simulink model "TesteEloGhendy"  (R2021b)
settings: Solver=FixedStepAuto  StartTime=0.0  StopTime=TempoSimulacao  RelTol=1e-3
values from neighbouring files (symbols this model uses):
  FatorSimulacao = 1e-3    (= 0.001)    [TesteRealCurtoFuses.m]    (also in TesteRealCurto_SemFuse.m)
  le = 1e-10    [TesteRealCurto.m]    (also in TesteRealCurtoFuses.m; TesteRealCurto_SemFuse.m)
  lm = (imag(Zm)/(2*pi*f))*d    [TesteRealCurto.m]    (also in TesteRealCurtoFuses.m; TesteRealCurto_SemFuse.m)
  lp = (imag(Zp)/(2*pi*f))*d    [TesteRealCurto.m]    (also in TesteRealCurtoFuses.m; TesteRealCurto_SemFuse.m)
  NRE = 1e-12    [TesteRealCurto.m]    (also in TesteRealCurtoFuses.m; TesteRealCurto_SemFuse.m)
  rm = real(Zm)*d    [TesteRealCurto.m]    (also in TesteRealCurtoFuses.m; TesteRealCurto_SemFuse.m)
  rp = real(Zp)*d    [TesteRealCurto.m]    (also in TesteRealCurtoFuses.m; TesteRealCurto_SemFuse.m)
  rtc = 10    [TesteRealCurto.m]    (also in TesteRealCurtoFuses.m; TesteRealCurto_SemFuse.m)
  rti = 10    [TesteRealCurto.m]    (also in TesteRealCurtoFuses.m; TesteRealCurto_SemFuse.m)
undefined symbols (not defined in the file or in its folder): D11, Delta, POT, PotConsumidor, Ra_Curto, Rb_Curto, Rc_Curto
libraries: spsRMSLib x15, spsBreakerLib x7, spsCurrentMeasurementLib x7, spsSeriesRLCBranchLib x6, spsThreePhaseVIMeasurementLib x4, spsThreePhaseTransformerTwoWindingsLib x2, spsThreePhaseSeriesRLCLoadLib x1, spsThreePhaseBreakerLib x1, spsThreePhaseSourceLib x1, spsMutualInductanceLib x1, spspowerguiLib x1
(part 1 of 2)
settings Model: Creator=USER  LastModifiedBy=Leonardo-Felipe
settings SolverCC: ZeroCrossAlgorithm=Adaptive
settings DebuggingCC: MaskedZcDiagnostic=none  IgnoredZcDiagnostic=none

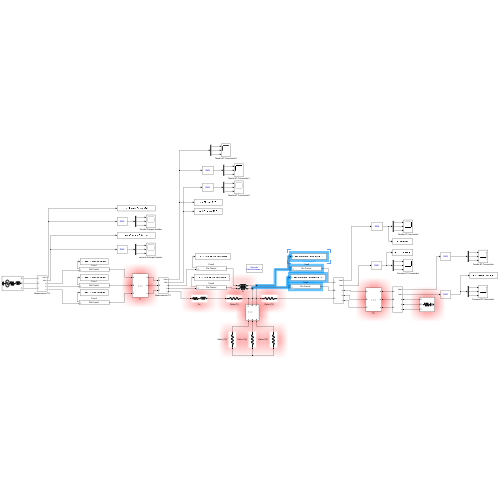
[thumbnail: Simulink's stored preview of the top-level diagram]
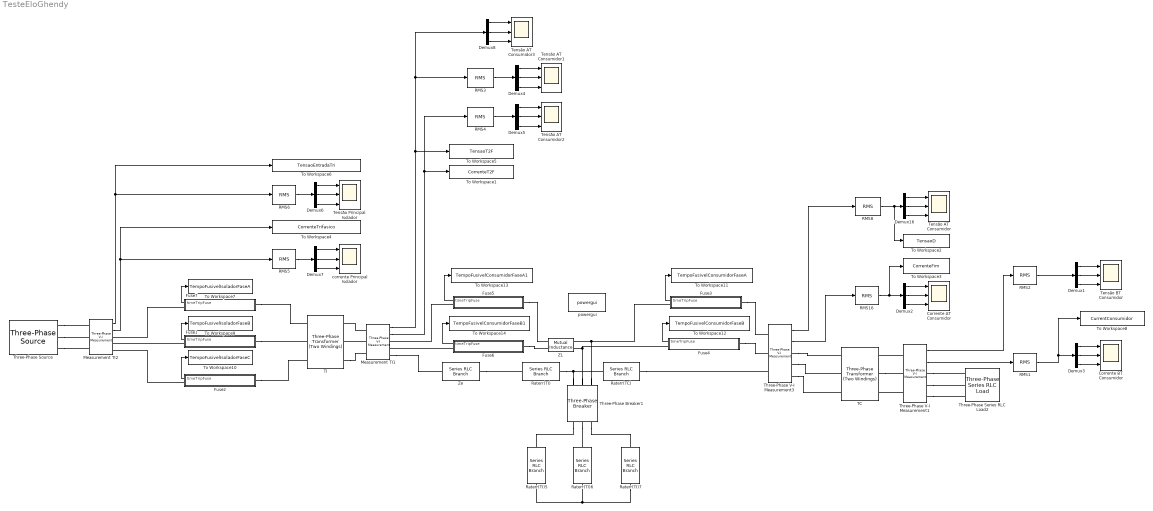
== system TesteEloGhendy ==
  Corrente AT Consumidor : Scope  NumInputPorts=3
  Corrente BT Consumidor : Scope  NumInputPorts=3
  Demux{1..8,16} (9 alike) : Demux  Outputs=3
  Fuse1 : Subsystem  mask{tipofuse=15K, a=346.4070, b=-257.6697, c=71.6644, d=-8.8225, e=0.4027, IoTot=15}
      mask prompts: tipofuse "Tipo de Fusivel"
      mask TypeOptions tipofuse: 15K
      mask Callback tipofuse:
      | switch(get_param(gcb,'tipofuse'))
      |     case '1H'
      |         set_param(gcb,'a','11.5834');
      |         set_param(gcb,'b','-7.7159');
      |         set_param(gcb,'c','2.2435');
      |         set_param(gcb,'d','-0.4141');
      |         set_param(gcb,'e','0.0293');
      |         set_param(gcb,'IoTot','1');
      |     case '2H'
      |         set_param(gcb,'a','15.3612');
      |         set_param(gcb,'b','-11.3048');
      |         set_param(gcb,'c','3.7855');
      |         set_param(gcb,'d','-0.6767');
      |         set_param(gcb,'e','0.0442');
      |         set_param(gcb,'IoTot','2');
      |     case '3H'
      |         set_param(gcb,'a','16.6469');
      |         set_param(gcb,'b','-10.3608');
      |         set_param(gcb,'c','2.8987');
      |         set_param(gcb,'d','-0.4844');
      |         set_param(gcb,'e','0.0315');
      |         set_param(gcb,'IoTot','3');
      |     case '5H'
      |         set_param(gcb,'a','33.5364');
      |         set_param(gcb,'b','-24.1389');
      |         set_param(gcb,'c','7.0071');
      |         set_param(gcb,'d','-1.0167');
      |         set_param(gcb,'e','0.0569');
      |         set_param(gcb,'IoTot','5');
      |     case '8H'
      |         set_param(gcb,'a','137.5572');
      |         set_param(gcb,'b','-119.0117');
      |         set_param(gcb,'c','38.2794');
      |         set_param(gcb,'d','-5.4440');
      |         set_param(gcb,'e','0.2846');
      |         set_param(gcb,'IoTot','8');
      |     case '6K'
      |         set_param(gcb,'a','181.2568');
      |         set_param(gcb,'b','-167.5711');
      |         set_param(gcb,'c','57.6673');
      |         set_param(gcb,'d','-8.7672');
      |         set_param(gcb,'e','0.4916');
      |         set_param(gcb,'IoTot','6');
      |     case '8K'
      |         set_param(gcb,'a','201.6778');
      |         set_param(gcb,'b','-175.2376');
      |         set_param(gcb,'c','56.8760');
      |         set_param(gcb,'d','-8.1725');
      |         set_param(gcb,'e','0.4340');
      |         set_param(gcb,'IoTot','8');
      |     case '10K'
      |         set_param(gcb,'a','251.8801');
      |         set_param(gcb,'b','-206.6378');
      |         set_param(gcb,'c','63.3069');
      |         set_param(gcb,'d','-8.5810');
      |         set_param(gcb,'e','0.4304');
      |         set_param(gcb,'IoTot','10');
      |     case '12K'
      |         set_param(gcb,'a','294.2461');
      |         set_param(gcb,'b','-229.0340');
      |         set_param(gcb,'c','66.6693');
      |         set_param(gcb,'d','-8.5945');
      |         set_param(gcb,'e','0.4107');
      |         set_param(gcb,'IoTot','12');
      |     case '15K'
      |         set_param(gcb,'a','346.4070');
      |         set_param(gcb,'b','-257.6697');
      |         set_param(gcb,'c','71.6644');
      |         set_param(gcb,'d','-8.8225');
      |         set_param(gcb,'e','0.4027');
      |         set_param(gcb,'IoTot','15');
      |     case '20K'
      |         set_param(gcb,'a','382.4620');
      |         set_param(gcb,'b','-271.3985');
      |         set_param(gcb,'c','72.1161');
      |         set_param(gcb,'d','-8.4924');
      |         set_param(gcb,'e','0.3714');
      |         set_param(gcb,'IoTot','20');
      |     case '25K'
      |         set_param(gcb,'a','469.9755');
      |         set_param(gcb,'b','-321.2512');
      |         set_param(gcb,'c','82.1749');
      |         set_param(gcb,'d','-9.3092');
      |         set_param(gcb,'e','0.3918');
      |         set_param(gcb,'IoTot','25');
      |     case '30K'
      |         set_param(gcb,'a','516.7220');
      |         set_param(gcb,'b','-337.6034');
      |         set_param(gcb,'c','82.5876');
      |         set_param(gcb,'d','-8.9522');
      |         set_param(gcb,'e','0.3608');
      |         set_param(gcb,'IoTot','30');
      |     case '40K'
      |         set_param(gcb,'a','672.1360');
      |         set_param(gcb,'b','-424.7867');
      |         set_param(gcb,'c','100.3706');
      |         set_param(gcb,'d','-10.4950');
      |         set_param(gcb,'e','0.4080');
      |         set_param(gcb,'IoTot','40');
      |     case '50K'
      |         set_param(gcb,'a','691.3953');
      |         set_param(gcb,'b','-419.2300');
      |         set_param(gcb,'c','95.1730');
      |         set_param(gcb,'d','-9.5735');
      |         set_param(gcb,'e','0.3584');
      |         set_param(gcb,'IoTot','50');
      |     case '65K'
      |         set_param(gcb,'a','841.8993');
      |         set_param(gcb,'b','-492.8148');
      |         set_param(gcb,'c','107.9499');
      |         set_param(gcb,'d','-10.4731');
      |         set_param(gcb,'e','0.3783');
      |         set_param(gcb,'IoTot','65');
      |     case '80K'
      |         set_param(gcb,'a','881.1649');
      |         set_param(gcb,'b','-499.4578');
      |         set_param(gcb,'c','106.0005');
      |         set_param(gcb,'d','-9.9685');
      |         set_param(gcb,'e','0.3492');
      |         set_param(gcb,'IoTot','80');
      |     case '100K'
      |         set_param(gcb,'a','1020.0325');
      |         set_param(gcb,'b','-554.4466');
      |         set_param(gcb,'c','112.8674');
      |         set_param(gcb,'d','-10.1845');
      |         set_param(gcb,'e','0.3425');
      |         set_param(gcb,'IoTot','100');
      | end
      mask Display: disp('Elo Fusivel');
  Fuse2 : Subsystem  mask{tipofuse=15K, a=346.4070, b=-257.6697, c=71.6644, d=-8.8225, e=0.4027, IoTot=15}
      mask prompts: tipofuse "Tipo de Fusivel"
      mask TypeOptions tipofuse: 15K
      mask Callback tipofuse:
      | switch(get_param(gcb,'tipofuse'))
      |     case '1H'
      |         set_param(gcb,'a','11.5834');
      |         set_param(gcb,'b','-7.7159');
      |         set_param(gcb,'c','2.2435');
      |         set_param(gcb,'d','-0.4141');
      |         set_param(gcb,'e','0.0293');
      |         set_param(gcb,'IoTot','1');
      |     case '2H'
      |         set_param(gcb,'a','15.3612');
      |         set_param(gcb,'b','-11.3048');
      |         set_param(gcb,'c','3.7855');
      |         set_param(gcb,'d','-0.6767');
      |         set_param(gcb,'e','0.0442');
      |         set_param(gcb,'IoTot','2');
      |     case '3H'
      |         set_param(gcb,'a','16.6469');
      |         set_param(gcb,'b','-10.3608');
      |         set_param(gcb,'c','2.8987');
      |         set_param(gcb,'d','-0.4844');
      |         set_param(gcb,'e','0.0315');
      |         set_param(gcb,'IoTot','3');
      |     case '5H'
      |         set_param(gcb,'a','33.5364');
      |         set_param(gcb,'b','-24.1389');
      |         set_param(gcb,'c','7.0071');
      |         set_param(gcb,'d','-1.0167');
      |         set_param(gcb,'e','0.0569');
      |         set_param(gcb,'IoTot','5');
      |     case '8H'
      |         set_param(gcb,'a','137.5572');
      |         set_param(gcb,'b','-119.0117');
      |         set_param(gcb,'c','38.2794');
      |         set_param(gcb,'d','-5.4440');
      |         set_param(gcb,'e','0.2846');
      |         set_param(gcb,'IoTot','8');
      |     case '6K'
      |         set_param(gcb,'a','181.2568');
      |         set_param(gcb,'b','-167.5711');
      |         set_param(gcb,'c','57.6673');
      |         set_param(gcb,'d','-8.7672');
      |         set_param(gcb,'e','0.4916');
      |         set_param(gcb,'IoTot','6');
      |     case '8K'
      |         set_param(gcb,'a','201.6778');
      |         set_param(gcb,'b','-175.2376');
      |         set_param(gcb,'c','56.8760');
      |         set_param(gcb,'d','-8.1725');
      |         set_param(gcb,'e','0.4340');
      |         set_param(gcb,'IoTot','8');
      |     case '10K'
      |         set_param(gcb,'a','251.8801');
      |         set_param(gcb,'b','-206.6378');
      |         set_param(gcb,'c','63.3069');
      |         set_param(gcb,'d','-8.5810');
      |         set_param(gcb,'e','0.4304');
      |         set_param(gcb,'IoTot','10');
      |     case '12K'
      |         set_param(gcb,'a','294.2461');
      |         set_param(gcb,'b','-229.0340');
      |         set_param(gcb,'c','66.6693');
      |         set_param(gcb,'d','-8.5945');
      |         set_param(gcb,'e','0.4107');
      |         set_param(gcb,'IoTot','12');
      |     case '15K'
      |         set_param(gcb,'a','346.4070');
      |         set_param(gcb,'b','-257.6697');
      |         set_param(gcb,'c','71.6644');
      |         set_param(gcb,'d','-8.8225');
      |         set_param(gcb,'e','0.4027');
      |         set_param(gcb,'IoTot','15');
      |     case '20K'
      |         set_param(gcb,'a','382.4620');
      |         set_param(gcb,'b','-271.3985');
      |         set_param(gcb,'c','72.1161');
      |         set_param(gcb,'d','-8.4924');
      |         set_param(gcb,'e','0.3714');
      |         set_param(gcb,'IoTot','20');
      |     case '25K'
      |         set_param(gcb,'a','469.9755');
      |         set_param(gcb,'b','-321.2512');
      |         set_param(gcb,'c','82.1749');
      |         set_param(gcb,'d','-9.3092');
      |         set_param(gcb,'e','0.3918');
      |         set_param(gcb,'IoTot','25');
      |     case '30K'
      |         set_param(gcb,'a','516.7220');
      |         set_param(gcb,'b','-337.6034');
      |         set_param(gcb,'c','82.5876');
      |         set_param(gcb,'d','-8.9522');
      |         set_param(gcb,'e','0.3608');
      |         set_param(gcb,'IoTot','30');
      |     case '40K'
      |         set_param(gcb,'a','672.1360');
      |         set_param(gcb,'b','-424.7867');
      |         set_param(gcb,'c','100.3706');
      |         set_param(gcb,'d','-10.4950');
      |         set_param(gcb,'e','0.4080');
      |         set_param(gcb,'IoTot','40');
      |     case '50K'
      |         set_param(gcb,'a','691.3953');
      |         set_param(gcb,'b','-419.2300');
      |         set_param(gcb,'c','95.1730');
      |         set_param(gcb,'d','-9.5735');
      |         set_param(gcb,'e','0.3584');
      |         set_param(gcb,'IoTot','50');
      |     case '65K'
      |         set_param(gcb,'a','841.8993');
      |         set_param(gcb,'b','-492.8148');
      |         set_param(gcb,'c','107.9499');
      |         set_param(gcb,'d','-10.4731');
      |         set_param(gcb,'e','0.3783');
      |         set_param(gcb,'IoTot','65');
      |     case '80K'
      |         set_param(gcb,'a','881.1649');
      |         set_param(gcb,'b','-499.4578');
      |         set_param(gcb,'c','106.0005');
      |         set_param(gcb,'d','-9.9685');
      |         set_param(gcb,'e','0.3492');
      |         set_param(gcb,'IoTot','80');
      |     case '100K'
      |         set_param(gcb,'a','1020.0325');
      |         set_param(gcb,'b','-554.4466');
      |         set_param(gcb,'c','112.8674');
      |         set_param(gcb,'d','-10.1845');
      |         set_param(gcb,'e','0.3425');
      |         set_param(gcb,'IoTot','100');
      | end
      mask Display: disp('Elo Fusivel');
  Fuse3 : Subsystem  mask{tipofuse=15K, a=346.4070, b=-257.6697, c=71.6644, d=-8.8225, e=0.4027, IoTot=15}
      mask prompts: tipofuse "Tipo de Fusivel"
      mask TypeOptions tipofuse: 15K
      mask Callback tipofuse:
      | switch(get_param(gcb,'tipofuse'))
      |     case '1H'
      |         set_param(gcb,'a','11.5834');
      |         set_param(gcb,'b','-7.7159');
      |         set_param(gcb,'c','2.2435');
      |         set_param(gcb,'d','-0.4141');
      |         set_param(gcb,'e','0.0293');
      |         set_param(gcb,'IoTot','1');
      |     case '2H'
      |         set_param(gcb,'a','15.3612');
      |         set_param(gcb,'b','-11.3048');
      |         set_param(gcb,'c','3.7855');
      |         set_param(gcb,'d','-0.6767');
      |         set_param(gcb,'e','0.0442');
      |         set_param(gcb,'IoTot','2');
      |     case '3H'
      |         set_param(gcb,'a','16.6469');
      |         set_param(gcb,'b','-10.3608');
      |         set_param(gcb,'c','2.8987');
      |         set_param(gcb,'d','-0.4844');
      |         set_param(gcb,'e','0.0315');
      |         set_param(gcb,'IoTot','3');
      |     case '5H'
      |         set_param(gcb,'a','33.5364');
      |         set_param(gcb,'b','-24.1389');
      |         set_param(gcb,'c','7.0071');
      |         set_param(gcb,'d','-1.0167');
      |         set_param(gcb,'e','0.0569');
      |         set_param(gcb,'IoTot','5');
      |     case '8H'
      |         set_param(gcb,'a','137.5572');
      |         set_param(gcb,'b','-119.0117');
      |         set_param(gcb,'c','38.2794');
      |         set_param(gcb,'d','-5.4440');
      |         set_param(gcb,'e','0.2846');
      |         set_param(gcb,'IoTot','8');
      |     case '6K'
      |         set_param(gcb,'a','181.2568');
      |         set_param(gcb,'b','-167.5711');
      |         set_param(gcb,'c','57.6673');
      |         set_param(gcb,'d','-8.7672');
      |         set_param(gcb,'e','0.4916');
      |         set_param(gcb,'IoTot','6');
      |     case '8K'
      |         set_param(gcb,'a','201.6778');
      |         set_param(gcb,'b','-175.2376');
      |         set_param(gcb,'c','56.8760');
      |         set_param(gcb,'d','-8.1725');
      |         set_param(gcb,'e','0.4340');
      |         set_param(gcb,'IoTot','8');
      |     case '10K'
      |         set_param(gcb,'a','251.8801');
      |         set_param(gcb,'b','-206.6378');
      |         set_param(gcb,'c','63.3069');
      |         set_param(gcb,'d','-8.5810');
      |         set_param(gcb,'e','0.4304');
      |         set_param(gcb,'IoTot','10');
      |     case '12K'
      |         set_param(gcb,'a','294.2461');
      |         set_param(gcb,'b','-229.0340');
      |         set_param(gcb,'c','66.6693');
      |         set_param(gcb,'d','-8.5945');
      |         set_param(gcb,'e','0.4107');
      |         set_param(gcb,'IoTot','12');
      |     case '15K'
      |         set_param(gcb,'a','346.4070');
      |         set_param(gcb,'b','-257.6697');
      |         set_param(gcb,'c','71.6644');
      |         set_param(gcb,'d','-8.8225');
      |         set_param(gcb,'e','0.4027');
      |         set_param(gcb,'IoTot','15');
      |     case '20K'
      |         set_param(gcb,'a','382.4620');
      |         set_param(gcb,'b','-271.3985');
      |         set_param(gcb,'c','72.1161');
      |         set_param(gcb,'d','-8.4924');
      |         set_param(gcb,'e','0.3714');
      |         set_param(gcb,'IoTot','20');
      |     case '25K'
      |         set_param(gcb,'a','469.9755');
      |         set_param(gcb,'b','-321.2512');
      |         set_param(gcb,'c','82.1749');
      |         set_param(gcb,'d','-9.3092');
      |         set_param(gcb,'e','0.3918');
      |         set_param(gcb,'IoTot','25');
      |     case '30K'
      |         set_param(gcb,'a','516.7220');
      |         set_param(gcb,'b','-337.6034');
      |         set_param(gcb,'c','82.5876');
      |         set_param(gcb,'d','-8.9522');
      |         set_param(gcb,'e','0.3608');
      |         set_param(gcb,'IoTot','30');
      |     case '40K'
      |         set_param(gcb,'a','672.1360');
      |         set_param(gcb,'b','-424.7867');
      |         set_param(gcb,'c','100.3706');
      |         set_param(gcb,'d','-10.4950');
      |         set_param(gcb,'e','0.4080');
      |         set_param(gcb,'IoTot','40');
      |     case '50K'
      |         set_param(gcb,'a','691.3953');
      |         set_param(gcb,'b','-419.2300');
      |         set_param(gcb,'c','95.1730');
      |         set_param(gcb,'d','-9.5735');
      |         set_param(gcb,'e','0.3584');
      |         set_param(gcb,'IoTot','50');
      |     case '65K'
      |         set_param(gcb,'a','841.8993');
      |         set_param(gcb,'b','-492.8148');
      |         set_param(gcb,'c','107.9499');
      |         set_param(gcb,'d','-10.4731');
      |         set_param(gcb,'e','0.3783');
      |         set_param(gcb,'IoTot','65');
      |     case '80K'
      |         set_param(gcb,'a','881.1649');
      |         set_param(gcb,'b','-499.4578');
      |         set_param(gcb,'c','106.0005');
      |         set_param(gcb,'d','-9.9685');
      |         set_param(gcb,'e','0.3492');
      |         set_param(gcb,'IoTot','80');
      |     case '100K'
      |         set_param(gcb,'a','1020.0325');
      |         set_param(gcb,'b','-554.4466');
      |         set_param(gcb,'c','112.8674');
      |         set_param(gcb,'d','-10.1845');
      |         set_param(gcb,'e','0.3425');
      |         set_param(gcb,'IoTot','100');
      | end
      mask Display: disp('Elo Fusivel');
  Fuse4 : Subsystem  mask{tipofuse=15K, a=346.4070, b=-257.6697, c=71.6644, d=-8.8225, e=0.4027, IoTot=15}
      mask prompts: tipofuse "Tipo de Fusivel"
      mask TypeOptions tipofuse: 15K
      mask Callback tipofuse:
      | switch(get_param(gcb,'tipofuse'))
      |     case '1H'
      |         set_param(gcb,'a','11.5834');
      |         set_param(gcb,'b','-7.7159');
      |         set_param(gcb,'c','2.2435');
      |         set_param(gcb,'d','-0.4141');
      |         set_param(gcb,'e','0.0293');
      |         set_param(gcb,'IoTot','1');
      |     case '2H'
      |         set_param(gcb,'a','15.3612');
      |         set_param(gcb,'b','-11.3048');
      |         set_param(gcb,'c','3.7855');
      |         set_param(gcb,'d','-0.6767');
      |         set_param(gcb,'e','0.0442');
      |         set_param(gcb,'IoTot','2');
      |     case '3H'
      |         set_param(gcb,'a','16.6469');
      |         set_param(gcb,'b','-10.3608');
      |         set_param(gcb,'c','2.8987');
      |         set_param(gcb,'d','-0.4844');
      |         set_param(gcb,'e','0.0315');
      |         set_param(gcb,'IoTot','3');
      |     case '5H'
      |         set_param(gcb,'a','33.5364');
      |         set_param(gcb,'b','-24.1389');
      |         set_param(gcb,'c','7.0071');
      |         set_param(gcb,'d','-1.0167');
      |         set_param(gcb,'e','0.0569');
      |         set_param(gcb,'IoTot','5');
      |     case '8H'
      |         set_param(gcb,'a','137.5572');
      |         set_param(gcb,'b','-119.0117');
      |         set_param(gcb,'c','38.2794');
      |         set_param(gcb,'d','-5.4440');
      |         set_param(gcb,'e','0.2846');
      |         set_param(gcb,'IoTot','8');
      |     case '6K'
      |         set_param(gcb,'a','181.2568');
      |         set_param(gcb,'b','-167.5711');
      |         set_param(gcb,'c','57.6673');
      |         set_param(gcb,'d','-8.7672');
      |         set_param(gcb,'e','0.4916');
      |         set_param(gcb,'IoTot','6');
      |     case '8K'
      |         set_param(gcb,'a','201.6778');
      |         set_param(gcb,'b','-175.2376');
      |         set_param(gcb,'c','56.8760');
      |         set_param(gcb,'d','-8.1725');
      |         set_param(gcb,'e','0.4340');
      |         set_param(gcb,'IoTot','8');
      |     case '10K'
      |         set_param(gcb,'a','251.8801');
      |         set_param(gcb,'b','-206.6378');
      |         set_param(gcb,'c','63.3069');
      |         set_param(gcb,'d','-8.5810');
      |         set_param(gcb,'e','0.4304');
      |         set_param(gcb,'IoTot','10');
      |     case '12K'
      |         set_param(gcb,'a','294.2461');
      |         set_param(gcb,'b','-229.0340');
      |         set_param(gcb,'c','66.6693');
      |         set_param(gcb,'d','-8.5945');
      |         set_param(gcb,'e','0.4107');
      |         set_param(gcb,'IoTot','12');
      |     case '15K'
      |         set_param(gcb,'a','346.4070');
      |         set_param(gcb,'b','-257.6697');
      |         set_param(gcb,'c','71.6644');
      |         set_param(gcb,'d','-8.8225');
      |         set_param(gcb,'e','0.4027');
      |         set_param(gcb,'IoTot','15');
      |     case '20K'
      |         set_param(gcb,'a','382.4620');
      |         set_param(gcb,'b','-271.3985');
      |         set_param(gcb,'c','72.1161');
      |         set_param(gcb,'d','-8.4924');
      |         set_param(gcb,'e','0.3714');
      |         set_param(gcb,'IoTot','20');
      |     case '25K'
      |         set_param(gcb,'a','469.9755');
      |         set_param(gcb,'b','-321.2512');
      |         set_param(gcb,'c','82.1749');
      |         set_param(gcb,'d','-9.3092');
      |         set_param(gcb,'e','0.3918');
      |         set_param(gcb,'IoTot','25');
      |     case '30K'
      |         set_param(gcb,'a','516.7220');
      |         set_param(gcb,'b','-337.6034');
      |         set_param(gcb,'c','82.5876');
      |         set_param(gcb,'d','-8.9522');
      |         set_param(gcb,'e','0.3608');
      |         set_param(gcb,'IoTot','30');
      |     case '40K'
      |         set_param(gcb,'a','672.1360');
      |         set_param(gcb,'b','-424.7867');
      |         set_param(gcb,'c','100.3706');
      |         set_param(gcb,'d','-10.4950');
      |         set_param(gcb,'e','0.4080');
      |         set_param(gcb,'IoTot','40');
      |     case '50K'
      |         set_param(gcb,'a','691.3953');
      |         set_param(gcb,'b','-419.2300');
      |         set_param(gcb,'c','95.1730');
      |         set_param(gcb,'d','-9.5735');
      |         set_param(gcb,'e','0.3584');
      |         set_param(gcb,'IoTot','50');
      |     case '65K'
      |         set_param(gcb,'a','841.8993');
      |         set_param(gcb,'b','-492.8148');
      |         set_param(gcb,'c','107.9499');
      |         set_param(gcb,'d','-10.4731');
      |         set_param(gcb,'e','0.3783');
      |         set_param(gcb,'IoTot','65');
      |     case '80K'
      |         set_param(gcb,'a','881.1649');
      |         set_param(gcb,'b','-499.4578');
      |         set_param(gcb,'c','106.0005');
      |         set_param(gcb,'d','-9.9685');
      |         set_param(gcb,'e','0.3492');
      |         set_param(gcb,'IoTot','80');
      |     case '100K'
      |         set_param(gcb,'a','1020.0325');
      |         set_param(gcb,'b','-554.4466');
      |         set_param(gcb,'c','112.8674');
      |         set_param(gcb,'d','-10.1845');
      |         set_param(gcb,'e','0.3425');
      |         set_param(gcb,'IoTot','100');
      | end
      mask Display: disp('Elo Fusivel');
  Fuse5 : Subsystem  mask{tipofuse=15K, a=346.4070, b=-257.6697, c=71.6644, d=-8.8225, e=0.4027, IoTot=15}
      mask prompts: tipofuse "Tipo de Fusivel"
      mask TypeOptions tipofuse: 15K
      mask Callback tipofuse:
      | switch(get_param(gcb,'tipofuse'))
      |     case '1H'
      |         set_param(gcb,'a','11.5834');
      |         set_param(gcb,'b','-7.7159');
      |         set_param(gcb,'c','2.2435');
      |         set_param(gcb,'d','-0.4141');
      |         set_param(gcb,'e','0.0293');
      |         set_param(gcb,'IoTot','1');
      |     case '2H'
      |         set_param(gcb,'a','15.3612');
      |         set_param(gcb,'b','-11.3048');
      |         set_param(gcb,'c','3.7855');
      |         set_param(gcb,'d','-0.6767');
      |         set_param(gcb,'e','0.0442');
      |         set_param(gcb,'IoTot','2');
      |     case '3H'
      |         set_param(gcb,'a','16.6469');
      |         set_param(gcb,'b','-10.3608');
      |         set_param(gcb,'c','2.8987');
      |         set_param(gcb,'d','-0.4844');
      |         set_param(gcb,'e','0.0315');
      |         set_param(gcb,'IoTot','3');
      |     case '5H'
      |         set_param(gcb,'a','33.5364');
      |         set_param(gcb,'b','-24.1389');
      |         set_param(gcb,'c','7.0071');
      |         set_param(gcb,'d','-1.0167');
      |         set_param(gcb,'e','0.0569');
      |         set_param(gcb,'IoTot','5');
      |     case '8H'
      |         set_param(gcb,'a','137.5572');
      |         set_param(gcb,'b','-119.0117');
      |         set_param(gcb,'c','38.2794');
      |         set_param(gcb,'d','-5.4440');
      |         set_param(gcb,'e','0.2846');
      |         set_param(gcb,'IoTot','8');
      |     case '6K'
      |         set_param(gcb,'a','181.2568');
      |         set_param(gcb,'b','-167.5711');
      |         set_param(gcb,'c','57.6673');
      |         set_param(gcb,'d','-8.7672');
      |         set_param(gcb,'e','0.4916');
      |         set_param(gcb,'IoTot','6');
      |     case '8K'
      |         set_param(gcb,'a','201.6778');
      |         set_param(gcb,'b','-175.2376');
      |         set_param(gcb,'c','56.8760');
      |         set_param(gcb,'d','-8.1725');
      |         set_param(gcb,'e','0.4340');
      |         set_param(gcb,'IoTot','8');
      |     case '10K'
      |         set_param(gcb,'a','251.8801');
      |         set_param(gcb,'b','-206.6378');
      |         set_param(gcb,'c','63.3069');
      |         set_param(gcb,'d','-8.5810');
      |         set_param(gcb,'e','0.4304');
      |         set_param(gcb,'IoTot','10');
      |     case '12K'
      |         set_param(gcb,'a','294.2461');
      |         set_param(gcb,'b','-229.0340');
      |         set_param(gcb,'c','66.6693');
      |         set_param(gcb,'d','-8.5945');
      |         set_param(gcb,'e','0.4107');
      |         set_param(gcb,'IoTot','12');
      |     case '15K'
      |         set_param(gcb,'a','346.4070');
      |         set_param(gcb,'b','-257.6697');
      |         set_param(gcb,'c','71.6644');
      |         set_param(gcb,'d','-8.8225');
      |         set_param(gcb,'e','0.4027');
      |         set_param(gcb,'IoTot','15');
      |     case '20K'
      |         set_param(gcb,'a','382.4620');
      |         set_param(gcb,'b','-271.3985');
      |         set_param(gcb,'c','72.1161');
      |         set_param(gcb,'d','-8.4924');
      |         set_param(gcb,'e','0.3714');
      |         set_param(gcb,'IoTot','20');
      |     case '25K'
      |         set_param(gcb,'a','469.9755');
      |         set_param(gcb,'b','-321.2512');
      |         set_param(gcb,'c','82.1749');
      |         set_param(gcb,'d','-9.3092');
      |         set_param(gcb,'e','0.3918');
      |         set_param(gcb,'IoTot','25');
      |     case '30K'
      |         set_param(gcb,'a','516.7220');
      |         set_param(gcb,'b','-337.6034');
      |         set_param(gcb,'c','82.5876');
      |         set_param(gcb,'d','-8.9522');
      |         set_param(gcb,'e','0.3608');
      |         set_param(gcb,'IoTot','30');
      |     case '40K'
      |         set_param(gcb,'a','672.1360');
      |         set_param(gcb,'b','-424.7867');
      |         set_param(gcb,'c','100.3706');
      |         set_param(gcb,'d','-10.4950');
      |         set_param(gcb,'e','0.4080');
      |         set_param(gcb,'IoTot','40');
      |     case '50K'
      |         set_param(gcb,'a','691.3953');
      |         set_param(gcb,'b','-419.2300');
      |         set_param(gcb,'c','95.1730');
      |         set_param(gcb,'d','-9.5735');
      |         set_param(gcb,'e','0.3584');
      |         set_param(gcb,'IoTot','50');
      |     case '65K'
      |         set_param(gcb,'a','841.8993');
      |         set_param(gcb,'b','-492.8148');
      |         set_param(gcb,'c','107.9499');
      |         set_param(gcb,'d','-10.4731');
      |         set_param(gcb,'e','0.3783');
      |         set_param(gcb,'IoTot','65');
      |     case '80K'
      |         set_param(gcb,'a','881.1649');
      |         set_param(gcb,'b','-499.4578');
      |         set_param(gcb,'c','106.0005');
      |         set_param(gcb,'d','-9.9685');
      |         set_param(gcb,'e','0.3492');
      |         set_param(gcb,'IoTot','80');
      |     case '100K'
      |         set_param(gcb,'a','1020.0325');
      |         set_param(gcb,'b','-554.4466');
      |         set_param(gcb,'c','112.8674');
      |         set_param(gcb,'d','-10.1845');
      |         set_param(gcb,'e','0.3425');
      |         set_param(gcb,'IoTot','100');
      | end
      mask Display: disp('Elo Fusivel');
  Fuse6 : Subsystem  mask{tipofuse=15K, a=346.4070, b=-257.6697, c=71.6644, d=-8.8225, e=0.4027, IoTot=15}
      mask prompts: tipofuse "Tipo de Fusivel"
      mask TypeOptions tipofuse: 15K
      mask Callback tipofuse:
      | switch(get_param(gcb,'tipofuse'))
      |     case '1H'
      |         set_param(gcb,'a','11.5834');
      |         set_param(gcb,'b','-7.7159');
      |         set_param(gcb,'c','2.2435');
      |         set_param(gcb,'d','-0.4141');
      |         set_param(gcb,'e','0.0293');
      |         set_param(gcb,'IoTot','1');
      |     case '2H'
      |         set_param(gcb,'a','15.3612');
      |         set_param(gcb,'b','-11.3048');
      |         set_param(gcb,'c','3.7855');
      |         set_param(gcb,'d','-0.6767');
      |         set_param(gcb,'e','0.0442');
      |         set_param(gcb,'IoTot','2');
      |     case '3H'
      |         set_param(gcb,'a','16.6469');
      |         set_param(gcb,'b','-10.3608');
      |         set_param(gcb,'c','2.8987');
      |         set_param(gcb,'d','-0.4844');
      |         set_param(gcb,'e','0.0315');
      |         set_param(gcb,'IoTot','3');
      |     case '5H'
      |         set_param(gcb,'a','33.5364');
      |         set_param(gcb,'b','-24.1389');
      |         set_param(gcb,'c','7.0071');
      |         set_param(gcb,'d','-1.0167');
      |         set_param(gcb,'e','0.0569');
      |         set_param(gcb,'IoTot','5');
      |     case '8H'
      |         set_param(gcb,'a','137.5572');
      |         set_param(gcb,'b','-119.0117');
      |         set_param(gcb,'c','38.2794');
      |         set_param(gcb,'d','-5.4440');
      |         set_param(gcb,'e','0.2846');
      |         set_param(gcb,'IoTot','8');
      |     case '6K'
      |         set_param(gcb,'a','181.2568');
      |         set_param(gcb,'b','-167.5711');
      |         set_param(gcb,'c','57.6673');
      |         set_param(gcb,'d','-8.7672');
      |         set_param(gcb,'e','0.4916');
      |         set_param(gcb,'IoTot','6');
      |     case '8K'
      |         set_param(gcb,'a','201.6778');
      |         set_param(gcb,'b','-175.2376');
      |         set_param(gcb,'c','56.8760');
      |         set_param(gcb,'d','-8.1725');
      |         set_param(gcb,'e','0.4340');
      |         set_param(gcb,'IoTot','8');
      |     case '10K'
      |         set_param(gcb,'a','251.8801');
      |         set_param(gcb,'b','-206.6378');
      |         set_param(gcb,'c','63.3069');
      |         set_param(gcb,'d','-8.5810');
      |         set_param(gcb,'e','0.4304');
      |         set_param(gcb,'IoTot','10');
      |     case '12K'
      |         set_param(gcb,'a','294.2461');
      |         set_param(gcb,'b','-229.0340');
      |         set_param(gcb,'c','66.6693');
      |         set_param(gcb,'d','-8.5945');
      |         set_param(gcb,'e','0.4107');
      |         set_param(gcb,'IoTot','12');
      |     case '15K'
      |         set_param(gcb,'a','346.4070');
      |         set_param(gcb,'b','-257.6697');
      |         set_param(gcb,'c','71.6644');
      |         set_param(gcb,'d','-8.8225');
      |         set_param(gcb,'e','0.4027');
      |         set_param(gcb,'IoTot','15');
      |     case '20K'
      |         set_param(gcb,'a','382.4620');
      |         set_param(gcb,'b','-271.3985');
      |         set_param(gcb,'c','72.1161');
      |         set_param(gcb,'d','-8.4924');
      |         set_param(gcb,'e','0.3714');
      |         set_param(gcb,'IoTot','20');
      |     case '25K'
      |         set_param(gcb,'a','469.9755');
      |         set_param(gcb,'b','-321.2512');
      |         set_param(gcb,'c','82.1749');
      |         set_param(gcb,'d','-9.3092');
      |         set_param(gcb,'e','0.3918');
      |         set_param(gcb,'IoTot','25');
      |     case '30K'
      |         set_param(gcb,'a','516.7220');
      |         set_param(gcb,'b','-337.6034');
      |         set_param(gcb,'c','82.5876');
      |         set_param(gcb,'d','-8.9522');
      |         set_param(gcb,'e','0.3608');
      |         set_param(gcb,'IoTot','30');
      |     case '40K'
      |         set_param(gcb,'a','672.1360');
      |         set_param(gcb,'b','-424.7867');
      |         set_param(gcb,'c','100.3706');
      |         set_param(gcb,'d','-10.4950');
      |         set_param(gcb,'e','0.4080');
      |         set_param(gcb,'IoTot','40');
      |     case '50K'
      |         set_param(gcb,'a','691.3953');
      |         set_param(gcb,'b','-419.2300');
      |         set_param(gcb,'c','95.1730');
      |         set_param(gcb,'d','-9.5735');
      |         set_param(gcb,'e','0.3584');
      |         set_param(gcb,'IoTot','50');
      |     case '65K'
      |         set_param(gcb,'a','841.8993');
      |         set_param(gcb,'b','-492.8148');
      |         set_param(gcb,'c','107.9499');
      |         set_param(gcb,'d','-10.4731');
      |         set_param(gcb,'e','0.3783');
      |         set_param(gcb,'IoTot','65');
      |     case '80K'
      |         set_param(gcb,'a','881.1649');
      |         set_param(gcb,'b','-499.4578');
      |         set_param(gcb,'c','106.0005');
      |         set_param(gcb,'d','-9.9685');
      |         set_param(gcb,'e','0.3492');
      |         set_param(gcb,'IoTot','80');
      |     case '100K'
      |         set_param(gcb,'a','1020.0325');
      |         set_param(gcb,'b','-554.4466');
      |         set_param(gcb,'c','112.8674');
      |         set_param(gcb,'d','-10.1845');
      |         set_param(gcb,'e','0.3425');
      |         set_param(gcb,'IoTot','100');
      | end
      mask Display: disp('Elo Fusivel');
  Fuse7 : Subsystem  mask{tipofuse=15K, a=346.4070, b=-257.6697, c=71.6644, d=-8.8225, e=0.4027, IoTot=15}
      mask prompts: tipofuse "Tipo de Fusivel"
      mask TypeOptions tipofuse: 15K
      mask Callback tipofuse:
      | switch(get_param(gcb,'tipofuse'))
      |     case '1H'
      |         set_param(gcb,'a','11.5834');
      |         set_param(gcb,'b','-7.7159');
      |         set_param(gcb,'c','2.2435');
      |         set_param(gcb,'d','-0.4141');
      |         set_param(gcb,'e','0.0293');
      |         set_param(gcb,'IoTot','1');
      |     case '2H'
      |         set_param(gcb,'a','15.3612');
      |         set_param(gcb,'b','-11.3048');
      |         set_param(gcb,'c','3.7855');
      |         set_param(gcb,'d','-0.6767');
      |         set_param(gcb,'e','0.0442');
      |         set_param(gcb,'IoTot','2');
      |     case '3H'
      |         set_param(gcb,'a','16.6469');
      |         set_param(gcb,'b','-10.3608');
      |         set_param(gcb,'c','2.8987');
      |         set_param(gcb,'d','-0.4844');
      |         set_param(gcb,'e','0.0315');
      |         set_param(gcb,'IoTot','3');
      |     case '5H'
      |         set_param(gcb,'a','33.5364');
      |         set_param(gcb,'b','-24.1389');
      |         set_param(gcb,'c','7.0071');
      |         set_param(gcb,'d','-1.0167');
      |         set_param(gcb,'e','0.0569');
      |         set_param(gcb,'IoTot','5');
      |     case '8H'
      |         set_param(gcb,'a','137.5572');
      |         set_param(gcb,'b','-119.0117');
      |         set_param(gcb,'c','38.2794');
      |         set_param(gcb,'d','-5.4440');
      |         set_param(gcb,'e','0.2846');
      |         set_param(gcb,'IoTot','8');
      |     case '6K'
      |         set_param(gcb,'a','181.2568');
      |         set_param(gcb,'b','-167.5711');
      |         set_param(gcb,'c','57.6673');
      |         set_param(gcb,'d','-8.7672');
      |         set_param(gcb,'e','0.4916');
      |         set_param(gcb,'IoTot','6');
      |     case '8K'
      |         set_param(gcb,'a','201.6778');
      |         set_param(gcb,'b','-175.2376');
      |         set_param(gcb,'c','56.8760');
      |         set_param(gcb,'d','-8.1725');
      |         set_param(gcb,'e','0.4340');
      |         set_param(gcb,'IoTot','8');
      |     case '10K'
      |         set_param(gcb,'a','251.8801');
      |         set_param(gcb,'b','-206.6378');
      |         set_param(gcb,'c','63.3069');
      |         set_param(gcb,'d','-8.5810');
      |         set_param(gcb,'e','0.4304');
      |         set_param(gcb,'IoTot','10');
      |     case '12K'
      |         set_param(gcb,'a','294.2461');
      |         set_param(gcb,'b','-229.0340');
      |         set_param(gcb,'c','66.6693');
      |         set_param(gcb,'d','-8.5945');
      |         set_param(gcb,'e','0.4107');
      |         set_param(gcb,'IoTot','12');
      |     case '15K'
      |         set_param(gcb,'a','346.4070');
      |         set_param(gcb,'b','-257.6697');
      |         set_param(gcb,'c','71.6644');
      |         set_param(gcb,'d','-8.8225');
      |         set_param(gcb,'e','0.4027');
      |         set_param(gcb,'IoTot','15');
      |     case '20K'
      |         set_param(gcb,'a','382.4620');
      |         set_param(gcb,'b','-271.3985');
      |         set_param(gcb,'c','72.1161');
      |         set_param(gcb,'d','-8.4924');
      |         set_param(gcb,'e','0.3714');
      |         set_param(gcb,'IoTot','20');
      |     case '25K'
      |         set_param(gcb,'a','469.9755');
      |         set_param(gcb,'b','-321.2512');
      |         set_param(gcb,'c','82.1749');
      |         set_param(gcb,'d','-9.3092');
      |         set_param(gcb,'e','0.3918');
      |         set_param(gcb,'IoTot','25');
      |     case '30K'
      |         set_param(gcb,'a','516.7220');
      |         set_param(gcb,'b','-337.6034');
      |         set_param(gcb,'c','82.5876');
      |         set_param(gcb,'d','-8.9522');
      |         set_param(gcb,'e','0.3608');
      |         set_param(gcb,'IoTot','30');
      |     case '40K'
      |         set_param(gcb,'a','672.1360');
      |         set_param(gcb,'b','-424.7867');
      |         set_param(gcb,'c','100.3706');
      |         set_param(gcb,'d','-10.4950');
      |         set_param(gcb,'e','0.4080');
      |         set_param(gcb,'IoTot','40');
      |     case '50K'
      |         set_param(gcb,'a','691.3953');
      |         set_param(gcb,'b','-419.2300');
      |         set_param(gcb,'c','95.1730');
      |         set_param(gcb,'d','-9.5735');
      |         set_param(gcb,'e','0.3584');
      |         set_param(gcb,'IoTot','50');
      |     case '65K'
      |         set_param(gcb,'a','841.8993');
      |         set_param(gcb,'b','-492.8148');
      |         set_param(gcb,'c','107.9499');
      |         set_param(gcb,'d','-10.4731');
      |         set_param(gcb,'e','0.3783');
      |         set_param(gcb,'IoTot','65');
      |     case '80K'
      |         set_param(gcb,'a','881.1649');
      |         set_param(gcb,'b','-499.4578');
      |         set_param(gcb,'c','106.0005');
      |         set_param(gcb,'d','-9.9685');
      |         set_param(gcb,'e','0.3492');
      |         set_param(gcb,'IoTot','80');
      |     case '100K'
      |         set_param(gcb,'a','1020.0325');
      |         set_param(gcb,'b','-554.4466');
      |         set_param(gcb,'c','112.8674');
      |         set_param(gcb,'d','-10.1845');
      |         set_param(gcb,'e','0.3425');
      |         set_param(gcb,'IoTot','100');
      | end
      mask Display: disp('Elo Fusivel');
  Measurement TI1 : spsThreePhaseVIMeasurementLib/Three-Phase V-I Measurement  VoltageMeasurement=phase-to-phase  SetLabelV=off  LabelV=Vabc  Vpu=off  VpuLL=off  CurrentMeasurement=yes  SetLabelI=off  LabelI=Iabc  Ipu=off  Pbase=100e6  Vbase=500e3  OutputType=Complex  PhasorSimulation=off  PSBequivalent=0
  Measurement TI2 : spsThreePhaseVIMeasurementLib/Three-Phase V-I Measurement  VoltageMeasurement=phase-to-ground  SetLabelV=off  LabelV=Vabc  Vpu=off  VpuLL=off  CurrentMeasurement=yes  SetLabelI=off  LabelI=Iabc  Ipu=off  Pbase=100e6  Vbase=500e3  OutputType=Complex  PhasorSimulation=off  PSBequivalent=0
  RMS{1..6,8,16} (8 alike) : spsRMSLib/RMS  TrueRMS=on  Freq=60  RMSInit=0  Ts=0
  Raterr(TC) : spsSeriesRLCBranchLib/Series RLC Branch  LConnTagsString=__new0  RConnTagsString=__new0  BranchType=R  Resistance=rtc  Inductance=0  SetiL0=off  InitialCurrent=0  Capacitance=1e-6  Setx0=off  InitialVoltage=0  Measurements=None
  Raterr(TI) : spsSeriesRLCBranchLib/Series RLC Branch  LConnTagsString=__new0  RConnTagsString=__new0  BranchType=R  Resistance=rti  Inductance=0  SetiL0=off  InitialCurrent=0  Capacitance=1e-6  Setx0=off  InitialVoltage=0  Measurements=None
  Raterr(TI)5 : spsSeriesRLCBranchLib/Series RLC Branch  LConnTagsString=__new0  RConnTagsString=__new0  BranchType=R  Resistance=Rc_Curto  Inductance=0  SetiL0=off  InitialCurrent=0  Capacitance=1e-6  Setx0=off  InitialVoltage=0  Measurements=None
  Raterr(TI)6 : spsSeriesRLCBranchLib/Series RLC Branch  LConnTagsString=__new0  RConnTagsString=__new0  BranchType=R  Resistance=Rb_Curto  Inductance=0  SetiL0=off  InitialCurrent=0  Capacitance=1e-6  Setx0=off  InitialVoltage=0  Measurements=None
  Raterr(TI)7 : spsSeriesRLCBranchLib/Series RLC Branch  LConnTagsString=__new0  RConnTagsString=__new0  BranchType=R  Resistance=Ra_Curto  Inductance=0  SetiL0=off  InitialCurrent=0  Capacitance=1e-6  Setx0=off  InitialVoltage=0  Measurements=None
  TC : spsThreePhaseTransformerTwoWindingsLib/Three-Phase Transformer (Two Windings)  Winding1Connection=Delta (D11)  Winding2Connection=Yg  CoreType=Three single-phase transformers  SetSaturation=off  Hysteresis=off  DataFile='hysteresis'  SetInitialFlux=off  Measurements=None  UNITS=pu  NominalPower=[PotConsumidor , 60]  Winding1=[13800 0.0048118 0.018511]  Winding2=[380 0.0048119 0.018511]  Rm=5.801193266567229e+02*1000  Lm=8.409977380031759e+02*1000  L0=0.50001  Saturation=[0 0;0.0012545 0.01913;0.52272 0.024231]  InitialFluxes=[-0.284979809735545 0.823658984534059 -0.538679174795599]  BreakLoop=on  DiscreteSolver=Trapezoidal iterative  DataType=off  TransfoNumber=1
  TI : spsThreePhaseTransformerTwoWindingsLib/Three-Phase Transformer (Two Windings)  Winding1Connection=Delta (D11)  Winding2Connection=Y  CoreType=Three single-phase transformers  SetSaturation=off  Hysteresis=off  DataFile='hysteresis'  SetInitialFlux=off  Measurements=None  UNITS=pu  NominalPower=[POT , 60 ]  Winding1=[13800 0.0048119 0.018511]  Winding2=[13800 0.0048119 0.018511]  Rm=1.730769230769231e+03*1000  Lm=40.010686750359440*1000  L0=6.3145  Saturation=[0 0;0.0012545 0.01913;0.52272 0.024231]  InitialFluxes=[-0.824307916361155 0.868219880297686 -0.043911963260012]  BreakLoop=on  DiscreteSolver=Trapezoidal iterative  DataType=off  TransfoNumber=1
  Tensão AT Consumidor{,1..3} (4 alike) : Scope  NumInputPorts=3
  Tensão BT Consumidor : Scope  NumInputPorts=3
  Tensão Principal Isolador : Scope  NumInputPorts=3
  Three-Phase Series RLC Load2 : spsThreePhaseSeriesRLCLoadLib/Three-Phase Series RLC Load  LConnTagsString=A|B|C  Configuration=Y (grounded)  NominalVoltage=220  Vabc=[220 220 220]  Vabcp=[1e3 1e3 1e3]  NominalFrequency=60  UnbalancedPower=off  ActivePower=PotConsumidor  InductivePower=0  CapacitivePower=0  Pabc=[5e3 5e3 5e3]  QLabc=[100 100 100]  QCabc=[100 100 100]  Pabcp=[10e3 9e3 11e3]  QLabcp=[100 90 110]  QCabcp=[100 90 110]  Measurements=None  LoadType=constant Z
  Three-Phase V-I Measurement1 : spsThreePhaseVIMeasurementLib/Three-Phase V-I Measurement  VoltageMeasurement=phase-to-phase  SetLabelV=off  LabelV=Vabc  Vpu=off  VpuLL=off  CurrentMeasurement=yes  SetLabelI=off  LabelI=Iabc  Ipu=off  Pbase=100e6  Vbase=500e3  OutputType=Magnitude  PhasorSimulation=off  PSBequivalent=0
  Three-Phase V-I Measurement3 : spsThreePhaseVIMeasurementLib/Three-Phase V-I Measurement  VoltageMeasurement=phase-to-phase  SetLabelV=off  LabelV=Vabc  Vpu=off  VpuLL=off  CurrentMeasurement=yes  SetLabelI=off  LabelI=Iabc  Ipu=off  Pbase=100e6  Vbase=500e3  OutputType=Magnitude  PhasorSimulation=off  PSBequivalent=0
  Three-Phase Breaker1 : spsThreePhaseBreakerLib/Three-Phase Breaker  InitialState=open  SwitchA=on  SwitchB=on  SwitchC=on  SwitchTimes=tempoAberturaFechamento  External=off  BreakerResistance=0.01  SnubberResistance=1e6  SnubberCapacitance=inf  Measurements=None
  Three-Phase Source : spsThreePhaseSourceLib/Three-Phase Source  InternalConnection=Yg  VoltagePhases=off  Voltage=13.8e3  PhaseAngle=0  Voltage_phases=[25e3 25e3 25e3]/sqrt(3)  PhaseAngles_phases=[0 -120 +120]  Frequency=60  NonIdealSource=on  SpecifyImpedance=on  Resistance=0.8929  Inductance=16.58e-3  ShortCircuitLevel=120e6  BaseVoltage=13.8e3  XRratio=7  BusType=swing  Pref=10e3  Qref=0  Prefabc=[10e3, 10e3, 10e3]  Qrefabc=[0, 0, 0]  Qmin=-inf  Qmax=inf
  To Workspace1 : ToWorkspace  VariableName=CorrenteT2F  SampleTime=-1
  To Workspace10 : ToWorkspace  VariableName=TempoFusivelIsoladorFaseC  SampleTime=-1
      settings: MaxDataPoints=1  Save2DSignal=2-D array (concatenate along first dimension)
  To Workspace11 : ToWorkspace  VariableName=TempoFusivelConsumidorFaseA  SampleTime=-1
      settings: MaxDataPoints=1  Save2DSignal=2-D array (concatenate along first dimension)
  To Workspace12 : ToWorkspace  VariableName=TempoFusivelConsumidorFaseB  SampleTime=-1
      settings: MaxDataPoints=1  Save2DSignal=2-D array (concatenate along first dimension)
  To Workspace13 : ToWorkspace  VariableName=TempoFusivelConsumidorFaseA1  SampleTime=-1
      settings: MaxDataPoints=1  Save2DSignal=2-D array (concatenate along first dimension)
  To Workspace14 : ToWorkspace  VariableName=TempoFusivelConsumidorFaseB1  SampleTime=-1
      settings: MaxDataPoints=1  Save2DSignal=2-D array (concatenate along first dimension)
  To Workspace2 : ToWorkspace  VariableName=TensaoD  SampleTime=-1
  To Workspace3 : ToWorkspace  VariableName=CorrenteFim  SampleTime=-1
  To Workspace4 : ToWorkspace  VariableName=CorrenteTrifasico  SampleTime=-1
  To Workspace5 : ToWorkspace  VariableName=TensaoT2F  SampleTime=-1
  To Workspace6 : ToWorkspace  VariableName=TensaoEntradaTri  SampleTime=-1
  To Workspace7 : ToWorkspace  VariableName=TempoFusivelIsoladorFaseA  SampleTime=-1
      settings: MaxDataPoints=1  Save2DSignal=2-D array (concatenate along first dimension)
  To Workspace8 : ToWorkspace  VariableName=CurrentConsumidor  SampleTime=-1
  To Workspace9 : ToWorkspace  VariableName=TempoFusivelIsoladorFaseB  SampleTime=-1
      settings: MaxDataPoints=1  Save2DSignal=2-D array (concatenate along first dimension)
  ZL : spsMutualInductanceLib/Mutual Inductance  LConnTagsString=a|b  RConnTagsString=A|B  TypeOfMutual=Generalized mutual inductance  NumberOfWindings=2  SelfImpedance1=[1.1 1.1e-03]  SelfImpedance2=[ 1.1 1.1e-03]  ThreeWindings=on  SelfImpedance3=[ 1.1 1.1e-03]  MutualImpedance=[1.0 1.0e-03]  InductanceMatrix=[lp lm ; lm lp]  ResistanceMatrix=[rp rm ; rm rp]  Measurements=None
      settings: SourceProductBaseCode=PS
  Ze : spsSeriesRLCBranchLib/Series RLC Branch  LConnTagsString=__new0  RConnTagsString=__new0  BranchType=RL  Resistance=NRE  Inductance=le  SetiL0=off  InitialCurrent=0  Capacitance=le  Setx0=off  InitialVoltage=0  Measurements=None
  corrente Principal Isolador : Scope  NumInputPorts=3
  powergui : spspowerguiLib/powergui  Priority=1  SimulationMode=Discrete  SampleTime=FatorSimulacao  frequency=60  Iterations=50  frequencyindice=0  Pbase=100e6  ErrMax=1e-4  UnitsV=kV  UnitsW=MW  buscounter=0  FunctionMessages=on  echomessages=off  EnableUseOfTLC=on  CurrentSourceSwitches=on  DisableSnubberDevices=off  DisableRonSwitches=off  DisableVfSwitches=off  DisplayEquations=off  AutomaticDiscreteSolvers=on  SolverType=Tustin/Backward Euler (TBE)  Interpol=off  ExternalGateDelay=off  methode=off  Ts=100  x0status=blocks  SPID=on  SwTol=0  HookPort=off  NonlinearTolerance=1e-4  nMaxIteration=256  ContinueOnMaxIteration=off  RestoreLinks=warning  ResistiveCurrentMeasurement=off  Frange=[0:2:500]  Ylog=off  Xlog=on  ShowGrid=off  save=off  variable=ZData  structure=0  ZoomFFT=off  StartTime=0.0  cycles=1  DisplayStyle=1  fundamental=60  FreqAxis=off  MaxFrequency=1000  frequencyindicesteady=1  RmsSteady=1  display=off
  wires:
  Demux16/2 -> Tensão AT Consumidor/2
  Three-Phase V-I Measurement3/2 -> RMS16/1
  Demux16/3 -> Tensão AT Consumidor/3
  Demux16/1 -> Tensão AT Consumidor/1
  RMS8/1 -> Demux16/1, To Workspace2/1
  Three-Phase V-I Measurement3/1 -> RMS8/1
  Demux1/3 -> Tensão BT Consumidor/3
  RMS2/1 -> Demux1/1
  Demux1/1 -> Tensão BT Consumidor/1
  Demux1/2 -> Tensão BT Consumidor/2
  Demux2/3 -> Corrente AT Consumidor/3
  RMS16/1 -> To Workspace3/1, Demux2/1
  Demux2/1 -> Corrente AT Consumidor/1
  Demux2/2 -> Corrente AT Consumidor/2
  Demux3/2 -> Corrente BT Consumidor/2
  RMS1/1 -> Demux3/1, To Workspace8/1
  Demux3/1 -> Corrente BT Consumidor/1
  Demux3/3 -> Corrente BT Consumidor/3
  Measurement TI1/2 -> RMS4/1, To Workspace1/1
  RMS6/1 -> Demux6/1
  Demux6/3 -> Tensão Principal Isolador/3
  Demux7/1 -> corrente Principal Isolador/1
  RMS5/1 -> Demux7/1
  Demux7/3 -> corrente Principal Isolador/3
  Demux6/2 -> Tensão Principal Isolador/2
  Measurement TI2/1 -> To Workspace6/1, RMS6/1
  Demux6/1 -> Tensão Principal Isolador/1
  Demux7/2 -> corrente Principal Isolador/2
  Measurement TI2/2 -> To Workspace4/1, RMS5/1
  Three-Phase V-I Measurement1/1 -> RMS2/1
  Three-Phase V-I Measurement1/2 -> RMS1/1
  Fuse7/1(timeTripFuse) -> To Workspace7/1
  Fuse1/1(timeTripFuse) -> To Workspace9/1
  Fuse2/1(timeTripFuse) -> To Workspace10/1
  Fuse3/1(timeTripFuse) -> To Workspace11/1
  Fuse4/1(timeTripFuse) -> To Workspace12/1
  Fuse6/1(timeTripFuse) -> To Workspace14/1
  Fuse5/1(timeTripFuse) -> To Workspace13/1
  Demux4/1 -> Tensão AT Consumidor1/1
  Demux4/2 -> Tensão AT Consumidor1/2
  Demux4/3 -> Tensão AT Consumidor1/3
  RMS3/1 -> Demux4/1
  RMS4/1 -> Demux5/1
  Demux5/1 -> Tensão AT Consumidor2/1
  Demux5/2 -> Tensão AT Consumidor2/2
  Demux5/3 -> Tensão AT Consumidor2/3
  Demux8/3 -> Tensão AT Consumidor3/3
  Demux8/2 -> Tensão AT Consumidor3/2
  Demux8/1 -> Tensão AT Consumidor3/1
  Measurement TI1/1 -> Demux8/1, RMS3/1, To Workspace5/1
  connections:
  Three-Phase Breaker1/LConn1 -- Fuse3/RConn1 -- ZL/RConn1
  Raterr(TI)/RConn1 -- Raterr(TC)/LConn1 -- Three-Phase Breaker1/LConn3
  Three-Phase Breaker1/LConn2 -- Fuse4/RConn1 -- ZL/RConn2
  Three-Phase Source/RConn2 -- Measurement TI2/LConn2
  Measurement TI1/RConn3 -- Ze/LConn1
  Three-Phase Source/RConn3 -- Measurement TI2/LConn3
  Ze/RConn1 -- Raterr(TI)/LConn1
  Three-Phase Source/RConn1 -- Measurement TI2/LConn1
  Three-Phase V-I Measurement1/RConn2 -- Three-Phase Series RLC Load2/LConn2
  Three-Phase V-I Measurement1/RConn3 -- Three-Phase Series RLC Load2/LConn3
  Three-Phase V-I Measurement1/RConn1 -- Three-Phase Series RLC Load2/LConn1
  Raterr(TC)/RConn1 -- Three-Phase V-I Measurement3/LConn3
  Three-Phase V-I Measurement3/RConn1 -- TC/LConn1
  Three-Phase V-I Measurement3/RConn2 -- TC/LConn2
  Three-Phase V-I Measurement3/RConn3 -- TC/LConn3
  Three-Phase V-I Measurement1/LConn1 -- TC/RConn1
  Three-Phase V-I Measurement1/LConn3 -- TC/RConn3
  TC/RConn2 -- Three-Phase V-I Measurement1/LConn2
  Raterr(TI)7/RConn1 -- Raterr(TI)6/RConn1 -- Raterr(TI)5/RConn1
  Three-Phase Breaker1/RConn2 -- Raterr(TI)6/LConn1
  Three-Phase Breaker1/RConn3 -- Raterr(TI)5/LConn1
  Three-Phase Breaker1/RConn1 -- Raterr(TI)7/LConn1
  TI/RConn3 -- Measurement TI1/LConn3
  Measurement TI1/LConn2 -- TI/RConn2
  Measurement TI1/LConn1 -- TI/RConn1
  Fuse7/RConn1 -- Measurement TI2/RConn1
  Fuse7/LConn1 -- TI/LConn1
  Fuse2/LConn1 -- TI/LConn3
  Fuse1/LConn1 -- TI/LConn2
  Fuse1/RConn1 -- Measurement TI2/RConn2
  Fuse2/RConn1 -- Measurement TI2/RConn3
  Fuse4/LConn1 -- Three-Phase V-I Measurement3/LConn2
  Fuse3/LConn1 -- Three-Phase V-I Measurement3/LConn1
  Fuse6/LConn1 -- ZL/LConn2
  Fuse5/LConn1 -- ZL/LConn1
  Fuse5/RConn1 -- Measurement TI1/RConn1
  Fuse6/RConn1 -- Measurement TI1/RConn2
